simulink library "thc"  (R2021b)
settings: Solver=VariableStepAuto  StartTime=0.0  StopTime=10.0  RelTol=1e-3
undefined symbols (not defined in the file or in its folder): ATHC_APTCQA_X_C, ATHC_APTCQB_X_C, ATHC_dAy_X_C, ATHC_Qeq_X_kmh, ATHC_VbaseC_X_C, ATHC_VbaseC_Y_W, ATHC_VbaseD_X_C, ATHC_VbaseH_X_C, FALSE, KTHC_ACMaxMinT_sec, KTHC_aDeice_K, KTHC_AGSDefLv_K, KTHC_AGSLv1_K, KTHC_AGSLv2_K, KTHC_AGSLv3_K, KTHC_AGSLv4_K, KTHC_AGSLv5_K, KTHC_AirIntUpdateT_sec, KTHC_APTCOneZoneMax_W, KTHC_APTCPeriod_cnt, KTHC_APTCPWMEN_flg, KTHC_APTCQMaxC_W, KTHC_APTCQminC_W, KTHC_APTCQminD_W, KTHC_APTCQminRe1_W, KTHC_APTCQminRe_W, KTHC_APTCQoffT_cnt, KTHC_APTCQonT_cnt, KTHC_APTCRiLeMaxDff_W, KTHC_APTCRiLeMinDff_W, KTHC_BatInTempDef_C, KTHC_bDeice_K, KTHC_CompMaxDeice_rpm, KTHC_CompMinDeice_rpm, KTHC_CompSotxvOp_K, KTHC_CompSotxvOpLow_rpm, KTHC_CompSpdmax_rpm, KTHC_CompSpdmaxBC1_rpm, KTHC_CompSpdmaxBC_rpm, KTHC_CompSpdmid1_rpm, KTHC_CompSpdmid2_rpm, KTHC_CompSpdmid3_rpm, KTHC_CompSpdmid_rpm, KTHC_CompSpdmin_rpm, KTHC_DAPTCQ1_W, KTHC_DAPTCQ2_W, KTHC_DAPTCQ3_W, KTHC_DcChSetTemp_C, KTHC_DehumidityEN_flg, KTHC_DeiceCycTime_K, KTHC_DriveLevelWPTCBAH1_W, KTHC_DriveLevelWPTCBAH2_W, KTHC_DriveLevelWPTCBAH3_W, KTHC_DriveLevelWPTCBAH4_W, KTHC_DriveT1MinBAH_C, KTHC_DriveT2MaxBAH_C, KTHC_DriveT2MinBAH_C, KTHC_DriveT3MaxBAH_C, KTHC_DriveT3MinBAH_C, KTHC_DriveT4MaxBAH_C ... (+372)
libraries: simulink x140
(part 4 of 10)

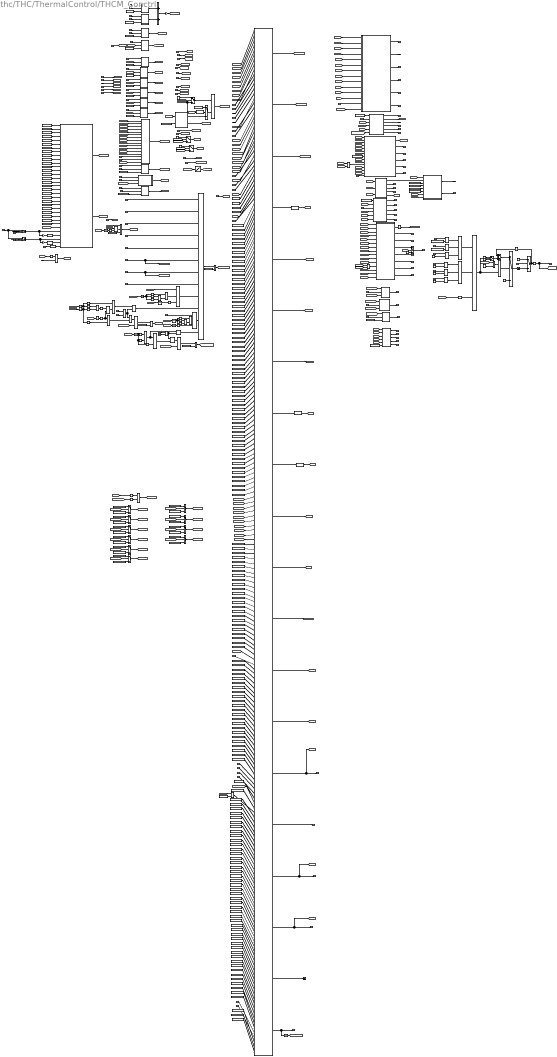
== system thc/THC/ThermalControl/THCM_Conctrl ==
  note: tick數 6000為10 min
  note: tick數 3000為5 min
  note: KTHC_DTcabin_C
  PwrSta : Inport
  AC : Inport  Port=2
  ACMax : Inport  Port=3
  ACAuto : Inport  Port=4
  sigSetTempZon1St : Inport  Port=5
  sigAirIntenZon1St : Inport  Port=6
  VehSpeed : Inport  Port=7
  HVBMTempMax : Inport  Port=8
  HVBMTempMin : Inport  Port=9
  OBCTemp : Inport  Port=10
  DCDCTemp : Inport  Port=11
  Rr_TMTemp : Inport  Port=12
  Rr_MCUTemp : Inport  Port=13
  Fr_TMTemp : Inport  Port=14
  Fr_MCUTemp : Inport  Port=15
  PT_ Low_P1 : Inport  Port=16
  PT_ Low_T1 : Inport  Port=17
  PT_Low_P2 : Inport  Port=18
  PT_ Low_T2 : Inport  Port=19
  PT_High_P : Inport  Port=20
  PT_High_Tact : Inport  Port=21
  Tamb : Inport  Port=22
  Bat_In_Temp : Inport  Port=23
  Bat_Out_Temp : Inport  Port=24
  Motor_In_Temp : Inport  Port=25
  Motor_Out_Temp : Inport  Port=26
  Tincar : Inport  Port=27
  SolarL : Inport  Port=28
  SolarR : Inport  Port=29
  Tevap : Inport  Port=30
  CompFB : Inport  Port=31
  CompProEN : Inport  Port=32
  VSCP_AGSCloseSta_flg : Inport  Port=33
  ShiftGearPosn : Inport  Port=34
  ChrgPlugSta : Inport  Port=35
  DfrstReq : Inport  Port=36
  WaterFillReq : Inport  Port=37
  sigSetTempZon2St : Inport  Port=38
  Fr_LLCTemp : Inport  Port=39
  Rr_LLCTemp : Inport  Port=40
  T_Face_L : Inport  Port=41
  T_Face_R : Inport  Port=42
  T_Foot_L : Inport  Port=43
  T_Foot_R : Inport  Port=44
  T_Face_Rr : Inport  Port=45
  T_Foot_Rr : Inport  Port=46
  PET : Inport  Port=47
  EACProtectEnable : Inport  Port=48
  Tamb_Err : Inport  Port=49
  SolarL_Err : Inport  Port=50
  SolarR_Err : Inport  Port=51
  Tevap_Err : Inport  Port=52
  T_Face_L_Err : Inport  Port=53
  T_Face_R_Err : Inport  Port=54
  T_Foot_L_Err : Inport  Port=55
  T_Foot_R_Err : Inport  Port=56
  T_Face_Rr_Err : Inport  Port=57
  T_Foot_Rr_Err : Inport  Port=58
  Tincar_Err : Inport  Port=59
  Bat_In_Temp_Err : Inport  Port=60
  Motor_In_Temp_Err : Inport  Port=61
  Motor_Out_Temp_Err : Inport  Port=62
  Fan_Err : Inport  Port=63
  AGS_Err : Inport  Port=64
  EWP3_Err : Inport  Port=65
  PT_High_P_Err : Inport  Port=66
  PT_High_Tact_Err : Inport  Port=67
  SOV1_Err : Inport  Port=68
  SOV2_Err : Inport  Port=69
  SOV3_Err : Inport  Port=70
  EXV1_Err : Inport  Port=71
  EXV2_Err : Inport  Port=72
  Comp_Err : Inport  Port=73
  Blower_Err : Inport  Port=74
  PT_Low_P1_Err : Inport  Port=75
  PT_Low_T1_Err : Inport  Port=76
  PT_Low_P2_Err : Inport  Port=77
  PT_Low_T2_Err : Inport  Port=78
  SOTXV_Err : Inport  Port=79
  ECOSW : Inport  Port=80
  RemoteACTemp : Inport  Port=81
  RemoteAutoReq : Inport  Port=82
  VINP_SmartEcoModeSW_flg : Inport  Port=83
  VINP_HVBIsoImpedenceN_Mohm : Inport  Port=84
  VINP_HVBIsoImpedenceP_Mohm : Inport  Port=85
  VINP_HVBHVILErr_flg : Inport  Port=86
  VINP_FrntPTCRearLeActHeatPwr_W : Inport  Port=87
  VINP_FrntPTCRearRiActHeatPwr_W : Inport  Port=88
  VINP_FrntPTCRiActHeatPwr_W : Inport  Port=89
  APTCFailDTC : Inport  Port=90
  RrAPTCEN : Inport  Port=91
  VINP_HVBattSOC_pct : Inport  Port=92
  VINP_IVIWPTCSWSta_flg : Inport  Port=93
  sigWindDirZon1St : Inport  Port=94
  1-D Lookup Table : Lookup_n-D  NumberOfTableDimensions=1  BreakpointsForDimension1=ATHC_dAy_X_C  Table=MTHC_dAy_Y_C  InternalRulePriority=Speed  RndMeth=Simplest  InputSameDT=on
  AGSandFan : Subsystem
  APTC : Subsystem
  Add1 : Sum
  Add2 : Sum
  BlowerCtrl : Subsystem
  Chart : Stateflow chart  TreatAsAtomicUnit=on
  Chart1 : Stateflow chart  TreatAsAtomicUnit=on
      settings: PortSchema="{\"entries\":[{\"content\":{\"sides\":[{\"content\":{\"connectorIds\":[\"In1\",\"In2\",\"In3\",\"In4\",\"In5\",\"In6\",\"In7\",\"In8\",\"In9\",\"In10\",\"In11\",\"In12\",\"In13\",\"In14\",\"In15\",\"In16\",\"In17\",\"In23\",\"In18\",\"In19\",\"In20\",\"In21\",\"In22\",\"In24\",\"In25\",\"In26\",\"In27\",\"In28\",\"In29\",\"In30\",\"In31\",\"In32\",\"In33\"]},\"type\":\"ConnectorPlacement.EquallySpacedRectSide\",\"uuid\":\"120e13ed-170d-4dd0-ac33-59229b58f73b\"},{\"content\":{\"connectorIds\":[\"Out1\",\"Out2\"],\"side\":\"RIGHT\"},\"type\":\"ConnectorPlacement.EquallySpacedRectSide\",\"uuid\":\"71523d45-f510-4724-888f-dcf7543ced53\"},{\"content\":{\"connectorIds\":[],\"side\":\"TOP\"},\"type\":\"ConnectorPlacement.EquallySpacedRectSide\",\"uuid\":\"9a401f36-06db-49d8-85fb-be71287fdb91\"}]},\"type\":\"ConnectorPlacement.EquallySpacedConnector\",\"uuid\":\"4c5defd4-093d-4cb1-85d3-718a50a7701f\"}],\"packageUris\":[\"http://schema.mathworks.com/mf0/Connector/R2020b\"],\"version\":\"1.0\"}"
  Chart2 : Stateflow chart  TreatAsAtomicUnit=on
  CompCtrl : Subsystem
  Compare To Constant : simulink/Logic and Bit Operations/Compare To Constant  relop=~=  const=1  OutDataTypeStr=boolean
  Compare To Constant1 : simulink/Logic and Bit Operations/Compare To Constant  relop=>  const=2  OutDataTypeStr=boolean
  Compare To Constant10 : simulink/Logic and Bit Operations/Compare To Constant  relop===  const=10  OutDataTypeStr=boolean
  Compare To Constant11 : simulink/Logic and Bit Operations/Compare To Constant  relop=~=  const=1  OutDataTypeStr=boolean
  Compare To Constant12 : simulink/Logic and Bit Operations/Compare To Constant  relop=>  const=2  OutDataTypeStr=boolean
  Compare To Constant13 : simulink/Logic and Bit Operations/Compare To Constant  relop=<  const=5  OutDataTypeStr=boolean
  Compare To Constant14 : simulink/Logic and Bit Operations/Compare To Constant  relop=<=  const=3.0  OutDataTypeStr=boolean
  Compare To Constant15 : simulink/Logic and Bit Operations/Compare To Constant  relop===  const=11  OutDataTypeStr=boolean
  Compare To Constant16 : simulink/Logic and Bit Operations/Compare To Constant  relop===  const=11  OutDataTypeStr=boolean
  Compare To Constant17 : simulink/Logic and Bit Operations/Compare To Constant  relop===  const=11  OutDataTypeStr=boolean
  Compare To Constant18 : simulink/Logic and Bit Operations/Compare To Constant  relop===  const=0  OutDataTypeStr=boolean
  Compare To Constant19 : simulink/Logic and Bit Operations/Compare To Constant  relop=>=  const=10  OutDataTypeStr=boolean
  Compare To Constant2 : simulink/Logic and Bit Operations/Compare To Constant  relop=<  const=10  OutDataTypeStr=boolean
  Compare To Constant20 : simulink/Logic and Bit Operations/Compare To Constant  relop=>  const=0  OutDataTypeStr=boolean
  Compare To Constant21 : simulink/Logic and Bit Operations/Compare To Constant  relop===  const=1  OutDataTypeStr=boolean
  Compare To Constant3 : simulink/Logic and Bit Operations/Compare To Constant  relop=>  const=7  OutDataTypeStr=boolean
  Compare To Constant4 : simulink/Logic and Bit Operations/Compare To Constant  relop=<  const=10  OutDataTypeStr=boolean
  Compare To Constant5 : simulink/Logic and Bit Operations/Compare To Constant  relop===  const=5  OutDataTypeStr=boolean
  Compare To Constant6 : simulink/Logic and Bit Operations/Compare To Constant  relop===  const=1  OutDataTypeStr=boolean
  Compare To Constant7 : simulink/Logic and Bit Operations/Compare To Constant  relop===  const=10  OutDataTypeStr=boolean
  Compare To Constant8 : simulink/Logic and Bit Operations/Compare To Constant  relop===  const=3  OutDataTypeStr=boolean
  Compare To Constant9 : simulink/Logic and Bit Operations/Compare To Constant  relop===  const=1  OutDataTypeStr=boolean
  Constant : Constant  Value=KTHC_T1MaxBC_C
  Constant1 : Constant  Value=KTHC_Plow2Setpoint_kPa
  Constant10 : Constant  Value=KTHC_T3MinBC_C
  Constant100 : Constant  Value=KTHC_Tdeheat2_C
  Constant101 : Constant  Value=KTHC_T1MinBAH_C
  Constant102 : Constant  Value=KTHC_CompMaxDeice_rpm
  Constant103 : Constant  Value=KTHC_CompMinDeice_rpm
  Constant104 : Constant  Value=KTHC_DeiceCycTime_K
  Constant105 : Constant  Value=KTHC_PDeiceMax_kPa
  Constant106 : Constant  Value=KTHC_TDeice1_C
  Constant107 : Constant  Value=KTHC_TDeice2_C
  Constant108 : Constant  Value=KTHC_TambHPmin_C
  Constant109 : Constant  Value=KTHC_Time0_K
  Constant11 : Constant  Value=KTHC_T3MaxBC_C
  Constant110 : Constant  Value=KTHC_TimeDeiceMax_K
  Constant111 : Constant  Value=KTHC_TwOhtOff_C
  Constant112 : Constant  Value=KTHC_TwOhtOn_C
  Constant113 : Constant  Value=KTHC_aDeice_K
  Constant114 : Constant  Value=KTHC_bDeice_K
  Constant115 : Constant  Value=KTHC_ta_K
  Constant116 : Constant  Value=KTHC_tb_K
  Constant117 : Constant  Value=KTHC_CompSotxvOpLow_rpm
  Constant118 : Constant  Value=KTHC_CompSotxvOp_K
  Constant119 : Constant  Value=KTHC_SotxvProHi_kPa
  Constant12 : Constant  Value=KTHC_T4MinBC_C
  Constant120 : Constant  Value=KTHC_SotxvProLo_kPa
  Constant121 : Constant  Value=KTHC_T1MaxLLC_C
  Constant122 : Constant  Value=KTHC_T2MinLLC_C
  Constant123 : Constant  Value=KTHC_T2MaxLLC_C
  Constant124 : Constant  Value=KTHC_T3MinLLC_C
  Constant125 : Constant  Value=KTHC_T3MaxLLC_C
  Constant126 : Constant  Value=KTHC_T4MinLLC_C
  Constant127 : Constant  Value=KTHC_T4MaxLLC_C
  Constant128 : Constant  Value=KTHC_T5MinLLC_C
  Constant129 : Constant  Value=KTHC_TDcChgBC_C
  Constant13 : Constant  Value=KTHC_EXV1SHSetpoint_K
  Constant130 : Constant  Value=KTHC_TambDef_C
  Constant131 : Constant  Value=KTHC_SolarDef_W
  Constant132 : Constant  Value=KTHC_SolarDef_W
  Constant133 : Constant  Value=KTHC_Tevap_C
  Constant{134..139} (6 alike) : Constant  Value=KTHC_TductDef_C
  Constant14 : Constant  Value=KTHC_T4MaxBC_C
  Constant140 : Constant  Value=KTHC_BatInTempDef_C
  Constant141 : Constant  Value=KTHC_MotorOutTempDef_C
  Constant142 : Constant  Value=KTHC_WPTCDef_W
  Constant143 : Constant  Value=KTHC_CompSpdmaxBC_rpm
  Constant{144..148} (5 alike) : Constant  Value=KTHC_ErrHandleEN_flg
  Constant149 : Constant  Value=17
  Constant15 : Constant  Value=KTHC_T5MinBC_C
  Constant150 : Constant  Value=32
  Constant151 : Constant  Value=32
  Constant152 : Constant  Value=KTHC_SolarDebounceT_sec
  Constant153 : Constant  Value=KTHC_DTcabin_C
  Constant154 : Constant  Value=KTHC_DTreturn1_C
  Constant155 : Constant  Value=KTHC_DTreturn_C
  Constant156 : Constant  Value=KTHC_ECOTambLV1_C
  Constant157 : Constant  Value=KTHC_ECOTambLV2_C
  Constant158 : Constant  Value=KTHC_ECOTambLV3_C
  Constant159 : Constant  Value=KTHC_ECOTambLV4_C
  Constant16 : Constant  Value=KTHC_T1MaxCCU_C
  Constant160 : Constant  Value=KTHC_ECOTambLVT_sec
  Constant161 : Constant  Value=KTHC_ECOalpha1_K
  Constant162 : Constant  Value=KTHC_ECOalpha2_K
  Constant163 : Constant  Value=KTHC_ECOalpha3_K
  Constant164 : Constant  Value=KTHC_ECOalpha4_K
  Constant165 : Constant  Value=KTHC_ECOalpha5_K
  Constant166 : Constant  Value=KTHC_ECObeta1_K
  Constant167 : Constant  Value=KTHC_ECObeta2_K
  Constant168 : Constant  Value=KTHC_ECObeta3_K
  Constant169 : Constant  Value=KTHC_ECObeta4_K
  Constant17 : Constant  Value=KTHC_T3MinCCU_C
  Constant170 : Constant  Value=KTHC_ECObeta5_K
  Constant171 : Constant  Value=KTHC_ECObeta6_K
  Constant172 : Constant  Value=KTHC_ECObeta7_K
  Constant173 : Constant  Value=KTHC_ECObeta8_K
  Constant174 : Constant  Value=KTHC_ECObeta9_K
  Constant175 : Constant  Value=KTHC_ECOalpha6_K
  Constant176 : Constant  Value=KTHC_ECOalpha7_K
  Constant177 : Constant  Value=KTHC_ECOalpha8_K
  Constant178 : Constant  Value=KTHC_ECOalpha9_K
  Constant179 : Constant  Value=KTHC_ECOTambLV5_C
  Constant18 : Constant  Value=KTHC_T3MaxCCU_C
  Constant180 : Constant  Value=KTHC_ECOTambLV6_C
  Constant181 : Constant  Value=KTHC_ECOTambLV7_C
  Constant182 : Constant  Value=KTHC_ECOTambLV8_C
  Constant183 : Constant  Value=KTHC_DTcabin1_C
  Constant184 : Constant  Value=KTHC_DTcabin2_C
  Constant185 : Constant  Value=KTHC_DTreturn3_C
  Constant186 : Constant  Value=KTHC_DTimeCD_K
  Constant187 : Constant  Value=KTHC_DTambSat1_C
  Constant188 : Constant  Value=KTHC_DTambSat2_C
  Constant189 : Constant  Value=KTHC_APTCQMaxC_W
  Constant19 : Constant  Value=KTHC_T4MinCCU_C
  Constant190 : Constant  Value=KTHC_DTreturn2_C
  Constant191 : Constant  Value=KTHC_DTcabin3_C
  Constant192 : Constant  Value=KTHC_DTcabin4_C
  Constant193 : Constant  Value=KTHC_DTcabin5_C
  Constant194 : Constant  Value=KTHC_DTcabin6_C
  Constant195 : Constant  Value=KTHC_DTimeCD1_K
  Constant196 : Constant  Value=KTHC_DTimeCD2_K
  Constant197 : Constant  Value=KTHC_TambACmode1_C
  Constant198 : Constant  Value=KTHC_TambACmode2_C
  Constant199 : Constant  Value=KTHC_TambACmode3_C
  Constant2 : Constant  Value=KTHC_Timehu1_K
  Constant20 : Constant  Value=KTHC_T4MaxCCU_C
  Constant200 : Constant  Value=KTHC_TambACmode4_C
  Constant201 : Constant  Value=KTHC_DTcabin7_C
  Constant202 : Constant  Value=KTHC_DTcabin9_C
  Constant203 : Constant  Value=KTHC_DTcabin10_C
  Constant204 : Constant  Value=KTHC_DTreturn6_C
  Constant205 : Constant  Value=KTHC_DTambSat5_C
  Constant206 : Constant  Value=KTHC_APTCQminRe1_W
  Constant207 : Constant  Value=KTHC_DTCabin11_C
  Constant208 : Constant  Value=KTHC_TambSetLow_C
  Constant209 : Constant  Value=KTHC_Tcoolmin_C
  Constant21 : Constant  Value=KTHC_T5MinCCU_C
  Constant210 : Constant  Value=KTHC_TimeRe1_sec
  Constant211 : Constant  Value=KTHC_TimeRe2_sec
  Constant212 : Constant  Value=KTHC_Trecymin_C
  Constant213 : Constant  Value=KTHC_WoWPTC_flg
  Constant214 : Constant  Value=KTHC_DTreturn7_C
  Constant215 : Constant  Value=KTHC_DTambsat3_C
  Constant216 : Constant  Value=KTHC_TambACmode5_C
  Constant217 : Constant  Value=KTHC_TambACmode6_C
  Constant218 : Constant  Value=KTHC_CompSpdmid1_rpm
  Constant219 : Constant  Value=KTHC_CompSpdmid2_rpm
  Constant22 : Constant  Value=KTHC_T2MinCCU_C
  Constant220 : Constant  Value=KTHC_CompSpdmid3_rpm
  Constant221 : Constant  Value=KTHC_DTcabin12_C
  Constant222 : Constant  Value=KTHC_CompSpdmaxBC1_rpm
  Constant223 : Constant  Value=KTHC_HVBIsoImpedenceLV_Mohm
  Constant224 : Constant  Value=KTHC_HVBIsoImpedenceLV_Mohm
  Constant{225..228,244} (5 alike) : Constant  Value=0
  Constant229 : Constant  Value=KTHC_DriveT1MinBAH_C
  Constant23 : Constant  Value=KTHC_T2MaxCCU_C
  Constant230 : Constant  Value=KTHC_T2MinBAH_C
  Constant231 : Constant  Value=KTHC_DriveT2MinBAH_C
  Constant232 : Constant  Value=KTHC_DriveT3MaxBAH_C
  Constant233 : Constant  Value=KTHC_DTambsat4_C
  Constant234 : Constant  Value=KTHC_TambACmode7_C
  Constant235 : Constant  OutDataTypeStr=uint8
  Constant236 : Constant  Value=0  OutDataTypeStr=uint8
  Constant237 : Constant  Value=0  OutDataTypeStr=uint8
  Constant238 : Constant  Value=0  OutDataTypeStr=uint8
  Constant239 : Constant  Value=10  OutDataTypeStr=uint8
  Constant24 : Constant  Value=KTHC_T1MaxMCU_C
  Constant240 : Constant  Value=KTHC_DriveT2MaxBAH_C
  Constant241 : Constant  Value=KTHC_DriveT4MaxBAH_C
  Constant242 : Constant  Value=KTHC_LevelWPTCBAH3_W
  Constant243 : Constant  Value=KTHC_DriveLevelWPTCBAH1_W
  Constant245 : Constant  Value=KTHC_LevelWPTCBAH4_W
  Constant246 : Constant  Value=KTHC_DriveLevelWPTCBAH4_W
  Constant247 : Constant  Value=KTHC_EWPBalanceSW_flg
  Constant248 : Constant  Value=KTHC_DTwBMoin3_C
  Constant249 : Constant  Value=KTHC_HeatingFactor_C
  Constant25 : Constant  Value=KTHC_T3MinMCU_C
  Constant250 : Constant  Value=KTHC_ForceLeaveCool_C
  Constant251 : Constant  Value=KTHC_ForceLeaveHeat_C
  Constant26 : Constant  Value=KTHC_T3MaxMCU_C
  Constant27 : Constant  Value=KTHC_T4MinMCU_C
  Constant28 : Constant  Value=KTHC_T4MaxMCU_C
  Constant29 : Constant  Value=KTHC_T5MinMCU_C
  Constant3 : Constant  Value=KTHC_Timehu2_K
  Constant30 : Constant  Value=KTHC_T2MinMCU_C
  Constant31 : Constant  Value=KTHC_T2MaxMCU_C
  Constant32 : Constant  Value=KTHC_T1MaxMT_C
  Constant33 : Constant  Value=KTHC_T3MinMT_C
  Constant34 : Constant  Value=KTHC_T3MaxMT_C
  Constant35 : Constant  Value=KTHC_T4MinMT_C
  Constant36 : Constant  Value=KTHC_T4MaxMT_C
  Constant37 : Constant  Value=KTHC_T5MinMT_C
  Constant38 : Constant  Value=KTHC_T2MinMT_C
  Constant39 : Constant  Value=KTHC_T2MaxMT_C
  Constant4 : Constant  Value=KTHC_EXV2SHSetpoint_K
  Constant40 : Constant  Value=KTHC_P3MinHi_kPa
  Constant41 : Constant  Value=KTHC_P3MaxHi_kPa
  Constant42 : Constant  Value=KTHC_P4MinHi_kPa
  Constant43 : Constant  Value=KTHC_P4MaxHi_kPa
  Constant44 : Constant  Value=KTHC_P5MinHi_kPa
  Constant45 : Constant  Value=KTHC_P2MaxHi_kPa
  Constant46 : Constant  Value=KTHC_P3MaxLo_kPa
  Constant47 : Constant  Value=KTHC_P3MinLo_kPa
  Constant48 : Constant  Value=KTHC_P4MaxLo_kPa
  Constant49 : Constant  Value=KTHC_P4MinLo_kPa
  Constant5 : Constant  Value=KTHC_Tice_C
  Constant50 : Constant  Value=KTHC_P5MaxLo_kPa
  Constant51 : Constant  Value=KTHC_P2MinLo_kPa
  Constant52 : Constant  Value=KTHC_TWVRcolPos_pct
  Constant53 : Constant  Value=KTHC_TwRcolOn_C
  Constant54 : Constant  Value=KTHC_TwRcolOff_C
  Constant55 : Constant  Value=KTHC_DTambSat_C
  Constant56 : Constant  Value=KTHC_VehSdFanOn_kph
  Constant57 : Constant  Value=KTHC_VehSdFanOff_kph
  Constant58 : Constant  Value=KTHC_VehSdAGS100_kph
  Constant59 : Constant  Value=KTHC_VehSdAGSCtrl_kph
  Constant6 : Constant  Value=KTHC_Tdeice_C
  Constant60 : Constant  Value=KTHC_T2MinBH_C
  Constant61 : Constant  Value=KTHC_T3MaxBH_C
  Constant62 : Constant  Value=KTHC_T3MinBH_C
  Constant63 : Constant  Value=KTHC_T4MaxBH_C
  Constant64 : Constant  Value=KTHC_T4MinBH_C
  Constant65 : Constant  Value=KTHC_T5MaxBH_C
  Constant66 : Constant  Value=KTHC_DriveT3MinBAH_C
  Constant67 : Constant  Value=KTHC_T3MaxBAH_C
  Constant68 : Constant  Value=KTHC_T3MinBAH_C
  Constant69 : Constant  Value=KTHC_T4MaxBAH_C
  Constant7 : Constant  Value=KTHC_APTCQminD_W
  Constant70 : Constant  Value=KTHC_T2MaxBAH_C
  Constant71 : Constant  Value=KTHC_LevelWPTCBAH1_W
  Constant72 : Constant  Value=KTHC_DriveLevelWPTCBAH2_W
  Constant73 : Constant  Value=KTHC_LevelWPTCBAH2_W
  Constant74 : Constant  Value=KTHC_TWinmax_C
  Constant75 : Constant  Value=KTHC_TWinmin_C
  Constant76 : Constant  Value=KTHC_DriveLevelWPTCBAH3_W
  Constant77 : Constant  Value=KTHC_T1MinBH_C
  Constant78 : Constant  Value=KTHC_T2MaxBH_C
  Constant79 : Constant  Value=KTHC_DTwBMoin1_C
  Constant8 : Constant  Value=KTHC_T2MinBC_C
  Constant80 : Constant  Value=KTHC_DTwBMoin2_C
  Constant81 : Constant  Value=KTHC_DTwBBin_C
  Constant82 : Constant  Value=KTHC_CompSpdmax_rpm
  Constant83 : Constant  Value=KTHC_TBPmax_C
  Constant84 : Constant  Value=KTHC_TBPmin_C
  Constant85 : Constant  Value=KTHC_T3winSetpointBC_C
  Constant86 : Constant  Value=KTHC_Timewcd_K
  Constant87 : Constant  Value=KTHC_CompSpdmin_rpm
  Constant88 : Constant  Value=KTHC_Plow2Setpoint_kPa
  Constant89 : Constant  Value=KTHC_DTh1_C
  Constant9 : Constant  Value=KTHC_T2MaxBC_C
  Constant90 : Constant  Value=KTHC_Tambset_C
  Constant91 : Constant  Value=KTHC_Twmset_C
  Constant92 : Constant  Value=KTHC_APTCQminRe_W
  Constant93 : Constant  Value=KTHC_CompSpdmid_rpm
  Constant94 : Constant  Value=KTHC_PhiDehum_kPa
  Constant95 : Constant  Value=KTHC_ThiDehum_C
  Constant96 : Constant  Value=KTHC_DehumidityEN_flg
  Constant97 : Constant  Value=KTHC_TimeD_K
  Constant98 : Constant  Value=KTHC_Tdefog_C
  Constant99 : Constant  Value=KTHC_Tdeheat1_C
  Data Type Conversion : DataTypeConversion  OutDataTypeStr=uint16
  Data Type Conversion1 : DataTypeConversion  OutDataTypeStr=uint16
  Data Type Conversion2 : DataTypeConversion  OutDataTypeStr=boolean
  EWP1 : Subsystem
  EWP2 : Subsystem
  EWP3 : Subsystem
  EXV1Ctrl : Subsystem
  EXV2Ctrl : Subsystem
  Gain : Gain  Gain=10
  Gain1 : Gain  Gain=10
  Gain2 : Gain  Gain=1/2
  Logical Operator{,12..13,31} (4 alike) : Logic  Inputs=3  AllPortsSameDT=off  OutDataTypeStr=boolean
  Logical Operator{1,3..5,10,14,17..18,25,27..28,32..33} (13 alike) : Logic  Operator=OR  AllPortsSameDT=off  OutDataTypeStr=boolean
  Logical Operator{2,6..7,9,11,15..16,19..24,26,35} (15 alike) : Logic  AllPortsSameDT=off  OutDataTypeStr=boolean
  Logical Operator29 : Logic  Operator=OR  Inputs=3  AllPortsSameDT=off  OutDataTypeStr=boolean
  Logical Operator30 : Logic  Operator=OR  Inputs=3  AllPortsSameDT=off  OutDataTypeStr=boolean
  Logical Operator8 : Logic  Operator=OR  Inputs=12  AllPortsSameDT=off  OutDataTypeStr=boolean
  NOT : Logic  Operator=NOT  IconShape=distinctive  AllPortsSameDT=off  OutDataTypeStr=boolean
  Product : Product
  RadiatorFan : Subsystem
  Relational Operator : RelationalOperator  Operator=<=  OutDataTypeStr=boolean  RndMeth=Simplest
  Relational Operator1 : RelationalOperator  Operator=<=  OutDataTypeStr=boolean  RndMeth=Simplest
  Relational Operator2 : RelationalOperator  Operator=~=  OutDataTypeStr=boolean  RndMeth=Simplest
  Relational Operator{3..5,7} (4 alike) : RelationalOperator  Operator=>  OutDataTypeStr=boolean  RndMeth=Simplest
  Saturation1 : Saturate  UpperLimit=10  LowerLimit=0
  Scope : Scope
  SensorErrorHandle1 : Subsystem
  SensorErrorHandle10 : Subsystem
  SensorErrorHandle11 : Subsystem
  SensorErrorHandle12 : Subsystem
  SensorErrorHandle2 : Subsystem
  SensorErrorHandle3 : Subsystem
  SensorErrorHandle4 : Subsystem
  SensorErrorHandle5 : Subsystem
  SensorErrorHandle6 : Subsystem
  SensorErrorHandle7 : Subsystem
  SensorErrorHandle8 : Subsystem
  SensorErrorHandle9 : Subsystem
  Subsystem : Subsystem
  Subsystem1 : Subsystem
  Subsystem2 : Subsystem
  Subsystem3 : Subsystem
  Subsystem4 : Subsystem
  Switch{,1..19} (20 alike) : Switch  Criteria=u2 > Threshold
  Thermal : Stateflow chart  TreatAsAtomicUnit=on
      settings: PortSchema="{\"entries\":[{\"content\":{\"sides\":[{\"content\":{\"connectorIds\":[\"In22\",\"In1\",\"In2\",\"In3\",\"In4\",\"In5\",\"In6\",\"In7\",\"In8\",\"In9\",\"In10\",\"In11\",\"In12\",\"In13\",\"In14\",\"In15\",\"In18\",\"In16\",\"In17\",\"In19\",\"In20\",\"In21\",\"In23\",\"In24\",\"In25\",\"In26\",\"In27\",\"In28\",\"In29\",\"In30\",\"In31\",\"In32\",\"In33\",\"In34\",\"In35\",\"In36\",\"In37\",\"In38\",\"In39\",\"In40\",\"In41\",\"In42\",\"In43\",\"In44\",\"In45\",\"In46\",\"In47\",\"In48\",\"In49\",\"In50\",\"In51\",\"In52\",\"In53\",\"In54\",\"In55\",\"In56\",\"In57\",\"In58\",\"In59\",\"In60\",\"In61\",\"In62\",\"In63\",\"In64\",\"In65\",\"In66\",\"In67\",\"In68\",\"In69\",\"In70\",\"In71\",\"In72\",\"In73\",\"In74\",\"In75\",\"In76\",\"In77\",\"In78\",\"In79\",\"In80\",\"In81\",\"In82\",\"In83\",\"In84\",\"In85\",\"In86\",\"In87\",\"In88\",\"In89\",\"In90\",\"In91\",\"In92\",\"In93\",\"In94\",\"In95\",\"In96\",\"In97\",\"In137\",\"In98\",\"In99\",\"In100\",\"In101\",\"In102\",\"In103\",\"In104\",\"In105\",\"In106\",\"In107\",\"In108\",\"In109\",\"In110\",\"In111\",\"In112\",\"In113\",\"In114\",\"In115\",\"In116\",\"In117\",\"In118\",\"In119\",\"In120\",\"In121\",\"In122\",\"In123\",\"In124\",\"In125\",\"In126\",\"In127\",\"In128\",\"In129\",\"In130\",\"In131\",\"In132\",\"In133\",\"In134\",\"In135\",\"In136\",\"In138\",\"In139\",\"In140\",\"In141\",\"In142\",\"In143\",\"In144\",\"In145\",\"In146\",\"In147\",\"In148\",\"In149\",\"In150\",\"In151\",\"In152\",\"In153\",\"In154\",\"In155\",\"In156\",\"In157\",\"In158\",\"In159\",\"In160\",\"In161\",\"In162\",\"In163\",\"In164\",\"In165\",\"In166\",\"In167\",\"In168\",\"In169\",\"In170\",\"In171\",\"In172\",\"In173\",\"In174\",\"In175\",\"In176\",\"In177\",\"In178\",\"In179\",\"In180\",\"In181\",\"In182\",\"In183\",\"In184\",\"In185\",\"In186\",\"In187\",\"In188\",\"In189\",\"In190\",\"In191\",\"In192\",\"In193\",\"In194\",\"In195\",\"In196\",\"In197\",\"In198\",\"In199\",\"In200\",\"In201\",\"In202\",\"In203\",\"In204\",\"In205\",\"In206\",\"In207\",\"In208\",\"In209\",\"In210\",\"In211\",\"In212\",\"In213\",\"In214\"]},\"type\":\"ConnectorPlacement.EquallySpacedRectSide\",\"uuid\":\"f0032f37-379c-4410-84d7-1f2e4d737994\"},{\"content\":{\"connectorIds\":[\"Out1\",\"Out2\",\"Out3\",\"Out4\",\"Out5\",\"Out6\",\"Out7\",\"Out8\",\"Out9\",\"Out10\",\"Out11\",\"Out12\",\"Out13\",\"Out14\",\"Out16\",\"Out18\",\"Out17\",\"Out15\",\"Out19\",\"Out20\"],\"side\":\"RIGHT\"},\"type\":\"ConnectorPlacement.EquallySpacedRectSide\",\"uuid\":\"1de0eec4-8da4-4f67-b701-80b707ee0866\"},{\"content\":{\"connectorIds\":[],\"side\":\"TOP\"},\"type\":\"ConnectorPlacement.EquallySpacedRectSide\",\"uuid\":\"b83953a5-08e8-430f-9593-9d2c74d0a81a\"}]},\"type\":\"ConnectorPlacement.EquallySpacedConnector\",\"uuid\":\"ef17bb72-69cc-4173-9cd7-5d5a49851498\"}],\"packageUris\":[\"http://schema.mathworks.com/mf0/Connector/R2020b\"],\"version\":\"1.0\"}"
  Unit Delay{,1..11} (12 alike) : UnitDelay  SampleTime=-1  HasFrameUpgradeWarning=on
  WPTC : Subsystem
  FD_Comp_Cmd : Outport
  FD_SOV1_Cmd : Outport  Port=2
  FD_SOV2_Cmd : Outport  Port=3
  FD_SOV3_Cmd : Outport  Port=4
  FD_EXV1_Cmd : Outport  Port=5
  FD_EXV2_Cmd : Outport  Port=6
  FD_SOTXV_Cmd : Outport  Port=7
  FD_FWV_Cmd : Outport  Port=8
  FD_TWV_Cmd : Outport  Port=9
  FD_FrWPTCHeatPwr_Cmd : Outport  Port=10
  CoolgFanActDuty : Outport  Port=11
  FD_AGS_Cmd : Outport  Port=12
  FD_EWP1_Cmd : Outport  Port=13
  FD_EWP2_Cmd : Outport  Port=14
  FD_EWP3_Cmd : Outport  Port=15
  FD_FrLeAPTCHeatPwr_Cmd : Outport  Port=16
  FD_FrRiAPTCHeatPwr_Cmd : Outport  Port=17
  FD_RrAPTCHeatPwr_Cmd : Outport  Port=18
  FD_Blower_Cmd : Outport  Port=19
  BatteryMode : Outport  Port=20
  EDriveMode : Outport  Port=21
  CabinMode : Outport  Port=22
  ACSubMode : Outport  Port=23
  VTHC_CompP_K : Outport  Port=24
  VTHC_CompI_K : Outport  Port=25
  VTHC_CompU_K : Outport  Port=26
  VTHC_CompDeltaU_K : Outport  Port=27
  VTHC_Compe_K : Outport  Port=28
  VTHC_Blowere_K : Outport  Port=29
  VTHC_BlowerP_K : Outport  Port=30
  VTHC_BlowerU_K : Outport  Port=31
  VTHC_Vbase_pct : Outport  Port=32
  VTHC_BlowerI_K : Outport  Port=33
  VTHC_EXV2P_K : Outport  Port=34
  VTHC_EXV2I_K : Outport  Port=35
  VTHC_EXV2U_K : Outport  Port=36
  VTHC_EXV2e_K : Outport  Port=37
  VTHC_APTCP_K : Outport  Port=38
  VTHC_APTCI_K : Outport  Port=39
  VTHC_APTCU_K : Outport  Port=40
  VTHC_APTCe_K : Outport  Port=41
  VTHC_EXV1P_K : Outport  Port=42
  VTHC_EXV1I_K : Outport  Port=43
  VTHC_EXV1U_K : Outport  Port=44
  VTHC_EXV1e_K : Outport  Port=45
  VTHC_FDCTHCMAPTCForceOFFSta_flg : Outport  Port=46
  VTHC_FDCTHCMPreWPTCHeatSta_enum : Outport  Port=47
  wires:
  Constant234/1 -> Thermal/209(KTHC_TambACmode7_C)
  Constant233/1 -> Thermal/208(KTHC_DTambsat4_C)
  [APTCForceOFF] -> Logical Operator33/2
  [ErrAPTCForceOFF] -> Logical Operator33/1
  Logical Operator33/1 -> APTC/12(ErrAPTCForceOFF)
  Logical Operator30/1 -> Logical Operator31/2
  Logical Operator29/1 -> Logical Operator31/1
  Relational Operator5/1 -> Logical Operator30/3
  Relational Operator4/1 -> Logical Operator30/2
  Relational Operator3/1 -> Logical Operator30/1
  Constant228/1 -> Relational Operator5/2
  VINP_FrntPTCRiActHeatPwr_W/1 -> Relational Operator5/1
  VINP_FrntPTCRearRiActHeatPwr_W/1 -> Relational Operator4/1
  Constant227/1 -> Relational Operator4/2
  Constant226/1 -> Relational Operator3/2
  VINP_FrntPTCRearLeActHeatPwr_W/1 -> Relational Operator3/1
  Relational Operator/1 -> Logical Operator29/1
  Relational Operator1/1 -> Logical Operator29/2
  Relational Operator2/1 -> Logical Operator29/3
  Constant225/1 -> Relational Operator2/2
  VINP_HVBHVILErr_flg/1 -> Relational Operator2/1
  Constant224/1 -> Relational Operator1/2
  VINP_HVBIsoImpedenceP_Mohm/1 -> Relational Operator1/1
  Constant223/1 -> Relational Operator/2
  VINP_HVBIsoImpedenceN_Mohm/1 -> Relational Operator/1
  Constant222/1 -> Thermal/207(KTHC_CompSpdmaxBC1_rpm)
  VINP_SmartEcoModeSW_flg/1 -> CompCtrl/15(VINP_SmartEcoModeSW_flg)
  Constant221/1 -> Thermal/206(KTHC_DTcabin12_C)
  Constant220/1 -> Thermal/205(KTHC_CompSpdmid3_rpm)
  Constant219/1 -> Thermal/204(KTHC_CompSpdmid2_rpm)
  Constant218/1 -> Thermal/203(KTHC_CompSpdmid1_rpm)
  [ACSubMode] -> Subsystem1/16(ACSubMode)
  Compare To Constant17/1 -> Logical Operator28/2
  Unit Delay9/1 -> Compare To Constant17/1
  [CabinMode] -> Unit Delay9/1
  Logical Operator28/1 -> Logical Operator13/2
  [AC] -> Logical Operator28/1
  Logical Operator27/1 -> Logical Operator12/2
  Compare To Constant16/1 -> Logical Operator27/1
  Logical Operator26/1 -> Logical Operator27/2
  Logical Operator25/1 -> Logical Operator/2
  Compare To Constant15/1 -> Logical Operator25/1
  Logical Operator24/1 -> Logical Operator25/2
  Constant217/1 -> Thermal/202(KTHC_TambACmode6_C)
  Constant216/1 -> Thermal/201(KTHC_TambACmode5_C)
  Constant215/1 -> Thermal/200(KTHC_DTambsat3_C)
  Constant214/1 -> Thermal/199(KTHC_DTreturn7_C)
  [PT_Low_P1] -> CompCtrl/14(PT_Low_P1)
  Constant213/1 -> Thermal/198(KTHC_WoWPTC_flg)
  [AC] -> APTC/15(AC)
  Data Type Conversion2/1 -> Chart1/33(ECOSW)
  Constant212/1 -> Thermal/197(KTHC_Trecymin_C)
  Constant211/1 -> Thermal/196(KTHC_TimeRe2_sec)
  Constant210/1 -> Thermal/195(KTHC_TimeRe1_sec)
  Constant209/1 -> Thermal/194(KTHC_Tcoolmin_C)
  Constant208/1 -> Thermal/193(KTHC_TambSetLow_C)
  Constant207/1 -> Thermal/192(KTHC_DTCabin11_C)
  Constant206/1 -> Thermal/191(KTHC_APTCQminRe1_W)
  [Tamb] -> APTC/14(Tamb)
  Constant205/1 -> Thermal/190(KTHC_DTambSat5_C)
  Constant204/1 -> Thermal/189(KTHC_DTreturn6_C)
  Constant203/1 -> Thermal/188(KTHC_DTcabin10_C)
  Constant202/1 -> Thermal/187(KTHC_DTcabin9_C)
  Thermal/1(AGS) -> [AGS]
  sigSetTempZon2St/1 -> Switch4/3
  sigSetTempZon1St/1 -> Switch3/3
  RemoteACTemp/1 -> Switch4/1, Switch3/1
  [Remote_AutoReq] -> Switch3/2
  [Remote_AutoReq] -> Switch4/2
  Compare To Constant14/1 -> Logical Operator23/1
  [PwrSta] -> Compare To Constant14/1
  Logical Operator23/1 -> [Remote_AutoReq]
  RemoteAutoReq/1 -> Logical Operator23/2
  Data Type Conversion1/1 -> Chart1/32(SetTempZon2St_CMD)
  Switch4/1 -> Chart1/31(sigSetTempZon2St), Gain1/1
  Gain1/1 -> Data Type Conversion1/1
  Data Type Conversion/1 -> Chart1/30(SetTempZon1St_CMD)
  Gain/1 -> Data Type Conversion/1
  Constant201/1 -> Thermal/186(KTHC_DTcabin7_C)
  Constant200/1 -> Thermal/185(KTHC_TambACmode4_C)
  Constant199/1 -> Thermal/184(KTHC_TambACmode3_C)
  Constant198/1 -> Thermal/183(KTHC_TambACmode2_C)
  Constant197/1 -> Thermal/182(KTHC_TambACmode1_C)
  Constant196/1 -> Thermal/181(KTHC_DTimeCD2_K)
  Constant195/1 -> Thermal/180(KTHC_DTimeCD1_K)
  Constant194/1 -> Thermal/179(KTHC_DTcabin6_C)
  Constant193/1 -> Thermal/178(KTHC_DTcabin5_C)
  Constant192/1 -> Thermal/177(KTHC_DTcabin4_C)
  Constant191/1 -> Thermal/176(KTHC_DTcabin3_C)
  Constant190/1 -> Thermal/175(KTHC_DTreturn2_C)
  Constant189/1 -> Thermal/174(KTHC_APTCQMaxC_W)
  [sigSetTempZon1StC] -> APTC/13(sigSetTempZon1StC)
  Constant188/1 -> Thermal/173(KTHC_DTambSat2_C)
  Constant187/1 -> Thermal/172(KTHC_DTambSat1_C)
  Constant185/1 -> Thermal/170(KTHC_DTreturn3_C)
  Constant186/1 -> Thermal/171(KTHC_DTimeCD_K)
  Constant184/1 -> Thermal/169(KTHC_DTcabin2_C)
  Constant183/1 -> Thermal/168(KTHC_DTcabin1_C)
  Constant182/1 -> Chart1/8(KTHC_ECOTambLV8_C)
  Constant181/1 -> Chart1/7(KTHC_ECOTambLV7_C)
  Constant180/1 -> Chart1/6(KTHC_ECOTambLV6_C)
  Constant179/1 -> Chart1/5(KTHC_ECOTambLV5_C)
  Constant178/1 -> Chart1/23(KTHC_ECOalpha9_K)
  Constant177/1 -> Chart1/17(KTHC_ECOalpha8_K)
  Constant176/1 -> Chart1/16(KTHC_ECOalpha7_K)
  Constant175/1 -> Chart1/15(KTHC_ECOalpha6_K)
  Constant174/1 -> Chart1/27(KTHC_ECObeta9_K)
  Constant173/1 -> Chart1/26(KTHC_ECObeta8_K)
  Constant172/1 -> Chart1/25(KTHC_ECObeta7_K)
  Constant171/1 -> Chart1/24(KTHC_ECObeta6_K)
  [sigSetTempZon2Stadj] -> Switch2/3
  [sigSetTempZon1Stadj] -> Switch1/3
  Chart1/2(sigSetTempZon2Stadj) -> [sigSetTempZon2Stadj]
  Chart1/1(sigSetTempZon1Stadj) -> [sigSetTempZon1Stadj]
  Constant170/1 -> Chart1/22(KTHC_ECObeta5_K)
  Constant169/1 -> Chart1/21(KTHC_ECObeta4_K)
  Constant168/1 -> Chart1/20(KTHC_ECObeta3_K)
  Constant167/1 -> Chart1/19(KTHC_ECObeta2_K)
  Constant166/1 -> Chart1/18(KTHC_ECObeta1_K)
  Constant165/1 -> Chart1/14(KTHC_ECOalpha5_K)
  Constant164/1 -> Chart1/13(KTHC_ECOalpha4_K)
  Constant163/1 -> Chart1/12(KTHC_ECOalpha3_K)
  Constant162/1 -> Chart1/11(KTHC_ECOalpha2_K)
  Constant161/1 -> Chart1/10(KTHC_ECOalpha1_K)
  Constant160/1 -> Chart1/9(KTHC_ECOTambLVT_sec)
  Constant159/1 -> Chart1/4(KTHC_ECOTambLV4_C)
  Constant158/1 -> Chart1/3(KTHC_ECOTambLV3_C)
  Constant157/1 -> Chart1/2(KTHC_ECOTambLV2_C)
  Constant156/1 -> Chart1/1(KTHC_ECOTambLV1_C)
  ECOSW/1 -> Data Type Conversion2/1
  [Tamb] -> Chart1/28(Tamb)
  Switch3/1 -> Chart1/29(sigSetTempZon1St), Gain/1
  Constant155/1 -> Thermal/167(KTHC_DTreturn_C)
  Constant154/1 -> Thermal/166(KTHC_DTreturn1_C)
  Constant153/1 -> Thermal/165(KTHC_DTcabin_C)
  Chart2/2(Blowersolar) -> [Blowersolar]
  Constant152/1 -> Chart2/2(KTHC_SolarDebounceT_sec)
  [sigSetTempZon2St] -> APTC/5(sigSetTempZon2St)
  [ACMax] -> Switch2/2
  Switch2/1 -> [sigSetTempZon2St]
  Constant151/1 -> Switch2/1
  Constant150/1 -> Switch1/1
  Switch1/1 -> [sigSetTempZon1St]
  [ACMax] -> Switch1/2
  Constant149/1 -> Switch/1
  [ACMax] -> Switch/2
  Switch/1 -> Product/1
  [sigSetTempZon1St] -> Subsystem4/1(sigSetTempZon1St), Switch/3
  [ACMax] -> Thermal/1(ACMax)
  ACMax/1 -> [ACMax]
  [Tamb_Err] -> Logical Operator22/1
  Logical Operator22/1 -> Thermal/164(Tamb_Err)
  Constant148/1 -> Logical Operator22/2
  Logical Operator21/1 -> [ErrEXV2FroceOFF]
  Logical Operator18/1 -> Logical Operator21/1
  Constant147/1 -> Logical Operator21/2
  Logical Operator17/1 -> Logical Operator20/1
  Logical Operator20/1 -> [ErrEXV1FroceOFF]
  Constant146/1 -> Logical Operator20/2
  Constant145/1 -> Logical Operator13/3
  Logical Operator8/1 -> Logical Operator19/1
  Logical Operator19/1 -> [ErrCompForceOFF]
  Constant144/1 -> Logical Operator19/2
  [Tamb] -> CompCtrl/13(Tamb)
  [Solar] -> Chart2/1(Solar)
  Chart2/1(FactorSolar) -> Switch19/3  "FactorSolar"
  Product/1 -> [sigSetTempZon1StC]
  [EXV2_Err] -> Logical Operator18/2
  [EXV1_Err] -> Logical Operator17/2
  Logical Operator16/1 -> Logical Operator18/1
  Logical Operator3/1 -> Logical Operator16/2
  Logical Operator12/1 -> Logical Operator8/11
  Logical Operator15/1 -> Logical Operator8/12
  [Tamb_Err] -> SensorErrorHandle12/2(SensorError)
  Tamb_Err/1 -> [Tamb_Err]
  Constant143/1 -> Thermal/163(KTHC_CompSpdmaxBC_rpm)
  [ErrCompForceOFF] -> Thermal/162(ErrCompForceOFF)
  [CompProEN] -> Logical Operator14/2
  [ErrCompForceOFF] -> Logical Operator14/1
  Logical Operator14/1 -> CompCtrl/11(CompProEN)
  Logical Operator13/1 -> [ErrAPTCForceOFF]
  [Blower_Err] -> Logical Operator13/1
  [AC] -> Thermal/22(AC)
  AC/1 -> [AC]
  [ErrEXV1FroceOFF] -> EXV1Ctrl/6(ErrEXV1FroceOFF)
  [ErrEXV2FroceOFF] -> EXV2Ctrl/6(ErrEXV2FroceOFF)
  SOTXV_Err/1 -> Logical Operator12/1
  Compare To Constant11/1 -> Logical Operator12/3
  Compare To Constant13/1 -> Logical Operator26/2
  Compare To Constant12/1 -> Logical Operator26/1
  Unit Delay8/1 -> Compare To Constant13/1, Compare To Constant12/1, Compare To Constant16/1
  [CabinMode] -> Unit Delay8/1
  [BatteryMode] -> Unit Delay7/1
  Unit Delay7/1 -> Compare To Constant11/1
  Logical Operator11/1 -> Logical Operator8/10
  Logical Operator10/1 -> Logical Operator11/1
  Logical Operator9/1 -> Logical Operator10/2
  Compare To Constant10/1 -> Logical Operator10/1
  Logical Operator5/1 -> Logical Operator6/2
  Logical Operator4/1 -> Logical Operator11/2, Logical Operator6/1
  NOT/1 -> Logical Operator9/1
  Unit Delay6/1 -> Compare To Constant9/1, Compare To Constant10/1
  Compare To Constant7/1 -> Logical Operator5/2
  Compare To Constant6/1 -> Logical Operator9/2, Logical Operator5/1
  Logical Operator7/1 -> NOT/1
  Logical Operator/1 -> Logical Operator8/9
  Comp_Err/1 -> Logical Operator8/8
  EXV2_Err/1 -> Logical Operator8/7, [EXV2_Err]
  EXV1_Err/1 -> Logical Operator8/6, [EXV1_Err]
  SOV3_Err/1 -> Logical Operator8/5
  SOV2_Err/1 -> Logical Operator8/4
  SOV1_Err/1 -> Logical Operator8/3
  PT_High_Tact_Err/1 -> Logical Operator8/2
  PT_High_P_Err/1 -> Logical Operator8/1
  Compare To Constant8/1 -> Logical Operator7/2
  Compare To Constant9/1 -> Logical Operator7/1
  Logical Operator6/1 -> Logical Operator17/1
  [ACSubMode] -> Unit Delay6/1
  [CabinMode] -> Unit Delay5/1
  Unit Delay5/1 -> Compare To Constant7/1, Compare To Constant8/1
  Unit Delay4/1 -> Compare To Constant6/1
  [BatteryMode] -> Unit Delay4/1
  PT_Low_T1_Err/1 -> Logical Operator4/2
  PT_Low_P1_Err/1 -> Logical Operator4/1
  PT_Low_T2_Err/1 -> Logical Operator1/2
  PT_Low_P2_Err/1 -> Logical Operator1/1
  Compare To Constant5/1 -> Logical Operator3/2
  Logical Operator2/1 -> Logical Operator3/1, Logical Operator15/1
  Compare To Constant4/1 -> Logical Operator2/2
  Compare To Constant3/1 -> Logical Operator2/1
  Logical Operator1/1 -> Logical Operator16/1, Logical Operator15/2
  Unit Delay3/1 -> Compare To Constant3/1, Compare To Constant4/1, Compare To Constant5/1
  [CabinMode] -> Unit Delay3/1
  [Blower_Err] -> Logical Operator/1
  Compare To Constant/1 -> Logical Operator/3
  Compare To Constant2/1 -> Logical Operator24/2
  Compare To Constant1/1 -> Logical Operator24/1
  Unit Delay/1 -> Compare To Constant1/1, Compare To Constant2/1, Compare To Constant15/1
  Unit Delay2/1 -> Compare To Constant/1
  [BatteryMode] -> Unit Delay2/1
  [CabinMode] -> Unit Delay/1
  Blower_Err/1 -> [Blower_Err]
  Constant142/1 -> WPTC/3(PresetValue)
  EWP3_Err/1 -> WPTC/2(EWP3_Err)
  [WPTC] -> WPTC/1(WPTC)
  Thermal/3(FrWPTCHeatPwr) -> [WPTC]  "FD_FrWPTCHeatPwr_Cmd"
  [AGS] -> RadiatorFan/3(AGS)
  AGS_Err/1 -> RadiatorFan/2(AGS_Err)
  [FAN] -> AGSandFan/3(FAN)
  Fan_Err/1 -> AGSandFan/2(Fan_Err)
  [FAN] -> RadiatorFan/1(FAN)
  [AGS] -> AGSandFan/1(AGSLV)
  Thermal/2(FAN) -> [FAN]
  Constant141/1 -> SensorErrorHandle11/3(PresetValue)
  Motor_Out_Temp_Err/1 -> SensorErrorHandle11/2(SensorError)
  Motor_Out_Temp/1 -> SensorErrorHandle11/1(DataIn)
  SensorErrorHandle11/1(DataOut) -> [Motor_Out_Temp]
  [TBMax] -> Subsystem2/3(TBMax)
  Motor_In_Temp_Err/1 -> Subsystem2/2(Motor_In_Temp_Err)
  Motor_In_Temp/1 -> Subsystem2/1(Motor_In_Temp)
  Subsystem2/1(Motor_In_TempFix) -> [Motor_In_Temp]
  [Motor_Out_Temp] -> Thermal/5(Motor_Out_Temp)
  [Motor_In_Temp] -> Thermal/4(Motor_In_Temp)
  Constant140/1 -> SensorErrorHandle10/3(PresetValue)
  SensorErrorHandle10/1(DataOut) -> [Bat_In_Temp]
  Bat_In_Temp_Err/1 -> SensorErrorHandle10/2(SensorError)
  Bat_In_Temp/1 -> SensorErrorHandle10/1(DataIn)
  Tincar_Err/1 -> Subsystem1/15(Tincar_Err)
  Tincar/1 -> Subsystem1/14(Tincar)
  [CabinMode] -> Subsystem1/13(CabinMode)
  Subsystem1/1(TincarFix) -> [Tincar]
  [T_Foot_Rr_Err] -> Subsystem1/12(T_Foot_Rr_Err)
  [T_Foot_Rr] -> Subsystem1/6(T_Foot_Rr)
  [T_Face_Rr] -> Subsystem1/5(T_Face_Rr)
  [T_Foot_R] -> Subsystem1/4(T_Foot_R)
  [T_Face_Rr_Err] -> Subsystem1/11(T_Face_Rr_Err)
  [T_Face_L] -> Subsystem1/1(T_Face_L)
  [T_Foot_R_Err] -> Subsystem1/10(T_Foot_R_Err)
  [T_Face_L_Err] -> Subsystem1/7(T_Face_L_Err)
  [T_Face_R] -> Subsystem1/2(T_Face_R)
  [T_Foot_L] -> Subsystem1/3(T_Foot_L)
  [T_Foot_L_Err] -> Subsystem1/9(T_Foot_L_Err)
  [T_Face_R_Err] -> Subsystem1/8(T_Face_R_Err)
  [T_Foot_Rr_Err] -> SensorErrorHandle9/2(SensorError)
  [T_Face_Rr_Err] -> SensorErrorHandle8/2(SensorError)
  [T_Foot_R_Err] -> SensorErrorHandle7/2(SensorError)
  [T_Foot_L_Err] -> SensorErrorHandle6/2(SensorError)
  [T_Face_R_Err] -> SensorErrorHandle5/2(SensorError)
  [T_Face_L_Err] -> SensorErrorHandle4/2(SensorError)
  SensorErrorHandle9/1(DataOut) -> [T_Foot_Rr]
  SensorErrorHandle8/1(DataOut) -> [T_Face_Rr]
  SensorErrorHandle7/1(DataOut) -> [T_Foot_R]
  SensorErrorHandle6/1(DataOut) -> [T_Foot_L]
  SensorErrorHandle5/1(DataOut) -> [T_Face_R]
  SensorErrorHandle4/1(DataOut) -> [T_Face_L]
  T_Foot_Rr/1 -> SensorErrorHandle9/1(DataIn)
  T_Face_Rr/1 -> SensorErrorHandle8/1(DataIn)
  T_Foot_R/1 -> SensorErrorHandle7/1(DataIn)
  T_Foot_L/1 -> SensorErrorHandle6/1(DataIn)
  T_Face_R/1 -> SensorErrorHandle5/1(DataIn)
  T_Face_L/1 -> SensorErrorHandle4/1(DataIn)
  Constant139/1 -> SensorErrorHandle9/3(PresetValue)
  Constant138/1 -> SensorErrorHandle8/3(PresetValue)
  Constant137/1 -> SensorErrorHandle7/3(PresetValue)
  Constant136/1 -> SensorErrorHandle6/3(PresetValue)
  Constant135/1 -> SensorErrorHandle5/3(PresetValue)
  Constant134/1 -> SensorErrorHandle4/3(PresetValue)
  T_Foot_Rr_Err/1 -> [T_Foot_Rr_Err]
  T_Face_Rr_Err/1 -> [T_Face_Rr_Err]
  T_Foot_R_Err/1 -> [T_Foot_R_Err]
  T_Foot_L_Err/1 -> [T_Foot_L_Err]
  T_Face_R_Err/1 -> [T_Face_R_Err]
  T_Face_L_Err/1 -> [T_Face_L_Err]
  [T_Foot_Rr] -> APTC/11(T_Foot_Rr)
  [T_Face_Rr] -> APTC/10(T_Face_Rr)
  [T_Foot_R] -> APTC/9(T_Foot_R)
  [T_Foot_L] -> APTC/8(T_Foot_L)
  [T_Face_R] -> APTC/7(T_Face_R)
  [T_Face_L] -> APTC/6(T_Face_L)
  [Tevap] -> Thermal/16(Tevap)
  SensorErrorHandle3/1(DataOut) -> [Tevap]
  Constant133/1 -> SensorErrorHandle3/3(PresetValue)
  Tevap_Err/1 -> SensorErrorHandle3/2(SensorError)
  Tevap/1 -> SensorErrorHandle3/1(DataIn)
  SensorErrorHandle2/1(DataOut) -> Add1/2
  SensorErrorHandle1/1(DataOut) -> Add1/1
  Constant132/1 -> SensorErrorHandle2/3(PresetValue)
  SolarR/1 -> SensorErrorHandle2/1(DataIn)
  SolarR_Err/1 -> SensorErrorHandle2/2(SensorError)
  Constant131/1 -> SensorErrorHandle1/3(PresetValue)
  SolarL_Err/1 -> SensorErrorHandle1/2(SensorError)
  SolarL/1 -> SensorErrorHandle1/1(DataIn)
  Constant130/1 -> SensorErrorHandle12/3(PresetValue)
  Tamb/1 -> SensorErrorHandle12/1(DataIn)
  SensorErrorHandle12/1(DataOut) -> [Tamb]
  Constant129/1 -> Thermal/161(KTHC_TDcChgBC_C)
  [EXVOpen] -> EXV2Ctrl/5(EXVOpen)
  [EXVOpen] -> EXV1Ctrl/5(EXVOpen)
  Subsystem/5(EXVOpen) -> [EXVOpen]
  EACProtectEnable/1 -> Thermal/160(EACProtectEnable)
  PET/1 -> Thermal/159(PET)
  Thermal/19(dy) -> Scope/1
  Rr_LLCTemp/1 -> Thermal/158(Rr_LLCTemp)
  Fr_LLCTemp/1 -> Thermal/157(Fr_LLCTemp)
  Constant128/1 -> Thermal/156(KTHC_T5MinLLC_C)
  Constant127/1 -> Thermal/155(KTHC_T4MaxLLC_C)
  Constant126/1 -> Thermal/154(KTHC_T4MinLLC_C)
  Constant125/1 -> Thermal/153(KTHC_T3MaxLLC_C)
  Constant124/1 -> Thermal/152(KTHC_T3MinLLC_C)
  Constant123/1 -> Thermal/151(KTHC_T2MaxLLC_C)
  Constant122/1 -> Thermal/150(KTHC_T2MinLLC_C)
  Constant121/1 -> Thermal/149(KTHC_T1MaxLLC_C)
  Thermal/12(SOTXV) -> [SOTXV]
  Constant118/1 -> Chart/4(KTHC_CompSotxvOp_K)
  Constant120/1 -> Chart/6(KTHC_SotxvProLo_kPa)
  Constant117/1 -> Chart/3(KTHC_CompSotxvOpLow_rpm)
  Constant119/1 -> Chart/5(KTHC_SotxvProHi_kPa)
  Subsystem/1(FD_Comp_Cmd) -> Chart/2(CompIn)
  [CabinMode] -> Chart/1(CabinMode)
  Chart/2(SOTXVout) -> FD_SOTXV_Cmd/1
  [PT_High_P] -> Chart/7(PT_High_P)
  [SOTXV] -> Chart/8(SOTXV)
  Constant116/1 -> Thermal/148(KTHC_tb_K)
  Constant115/1 -> Thermal/147(KTHC_ta_K)
  Constant114/1 -> Thermal/146(KTHC_bDeice_K)
  Constant113/1 -> Thermal/145(KTHC_aDeice_K)
  Constant112/1 -> Thermal/144(KTHC_TwOhtOn_C)
  Constant111/1 -> Thermal/143(KTHC_TwOhtOff_C)
  Constant110/1 -> Thermal/142(KTHC_TimeDeiceMax_K)
  Constant109/1 -> Thermal/141(KTHC_Time0_K)
  Constant108/1 -> Thermal/140(KTHC_TambHPmin_C)
  Constant107/1 -> Thermal/139(KTHC_TDeice2_C)
  Constant106/1 -> Thermal/138(KTHC_TDeice1_C)
  Constant105/1 -> Thermal/136(KTHC_PDeiceMax_kPa)
  Constant104/1 -> Thermal/135(KTHC_DeiceCycTime_K)
  Constant103/1 -> Thermal/134(KTHC_CompMinDeice_rpm)
  Constant102/1 -> Thermal/133(KTHC_CompMaxDeice_rpm)
  Bat_Out_Temp/1 -> Thermal/132(Bat_Out_Temp)
  [PwrSta] -> Thermal/7(PwrSta)
  [dAy] -> Thermal/131(dAy)
  1-D Lookup Table/1 -> [dAy]
  [Tamb] -> 1-D Lookup Table/1
  APTC/3(FD_FrRiAPTCHeatPwr_Cmd) -> FD_FrRiAPTCHeatPwr_Cmd/1  "FD_FrRiAPTCHeatPwr_Cmd"
  Switch11/1 -> FD_RrAPTCHeatPwr_Cmd/1  "FD_RrAPTCHeatPwr_Cmd"
  APTC/2(FD_FrLeAPTCHeatPwr_Cmd) -> FD_FrLeAPTCHeatPwr_Cmd/1  "FD_FrLeAPTCHeatPwr_Cmd"
  [VehSpeed] -> APTC/4(VehSpeed)
  [VehSpeed] -> Thermal/20(VehSpeed)
  Constant96/1 -> Thermal/130(KTHC_DehumidityEN_flg)
  Constant100/1 -> Thermal/129(KTHC_Tdeheat2_C)
  Constant99/1 -> Thermal/128(KTHC_Tdeheat1_C)
  Constant98/1 -> Thermal/127(KTHC_Tdefog_C)
  Constant97/1 -> Thermal/126(KTHC_TimeD_K)
  Constant95/1 -> Thermal/125(KTHC_ThiDehum_C)
  Constant94/1 -> Thermal/124(KTHC_PhiDehum_kPa)
  Constant93/1 -> Thermal/123(KTHC_CompSpdmid_rpm)
  Constant92/1 -> Thermal/122(KTHC_APTCQminRe_W)
  Constant91/1 -> Thermal/121(KTHC_Twmset_C)
  Constant90/1 -> Thermal/120(KTHC_Tambset_C)
  Constant89/1 -> Thermal/119(KTHC_DTh1_C)
  Constant88/1 -> Thermal/118(KTHC_Plow2Setpoint_kPa)
  Constant87/1 -> Thermal/117(KTHC_CompSpdmin_rpm)
  Constant86/1 -> Thermal/116(KTHC_Timewcd_K)
  Constant85/1 -> Thermal/115(KTHC_T3winSetpointBC_C)
  Constant84/1 -> Thermal/114(KTHC_TBPmin_C)
  Constant83/1 -> Thermal/113(KTHC_TBPmax_C)
  Constant82/1 -> Thermal/112(KTHC_CompSpdmax_rpm)
  Constant81/1 -> Thermal/111(KTHC_DTwBBin_C)
  Constant80/1 -> Thermal/110(KTHC_DTwBMoin2_C)
  Constant79/1 -> Thermal/109(KTHC_DTwBMoin1_C)
  Constant78/1 -> Thermal/91(KTHC_T2MaxBH_C)
  Constant77/1 -> Thermal/90(KTHC_T1MinBH_C)
  Constant75/1 -> Thermal/108(KTHC_TWinmin_C)
  Constant74/1 -> Thermal/107(KTHC_TWinmax_C)
  Constant65/1 -> Thermal/97(KTHC_T5MaxBH_C)
  Constant64/1 -> Thermal/96(KTHC_T4MinBH_C)
  Constant63/1 -> Thermal/95(KTHC_T4MaxBH_C)
  Constant62/1 -> Thermal/94(KTHC_T3MinBH_C)
  Constant61/1 -> Thermal/93(KTHC_T3MaxBH_C)
  Constant60/1 -> Thermal/92(KTHC_T2MinBH_C)
  Constant59/1 -> Thermal/89(KTHC_VehSdAGSCtrl_kph)
  Constant58/1 -> Thermal/88(KTHC_VehSdAGS100_kph)
  Constant57/1 -> Thermal/87(KTHC_VehSdFanOff_kph)
  Constant56/1 -> Thermal/86(KTHC_VehSdFanOn_kph)
  Constant55/1 -> Thermal/85(KTHC_DTambSat_C)
  Constant54/1 -> Thermal/84(KTHC_TwRcolOff_C)
  Constant53/1 -> Thermal/83(KTHC_TwRcolOn_C)
  Constant52/1 -> Thermal/82(KTHC_TWVRcolPos_pct)
  Constant50/1 -> Thermal/81(KTHC_P5MaxLo_kPa)
  Constant49/1 -> Thermal/80(KTHC_P4MinLo_kPa)
  Constant48/1 -> Thermal/79(KTHC_P4MaxLo_kPa)
  Constant47/1 -> Thermal/78(KTHC_P3MinLo_kPa)
  Constant46/1 -> Thermal/77(KTHC_P3MaxLo_kPa)
  Constant51/1 -> Thermal/76(KTHC_P2MinLo_kPa)
  Constant44/1 -> Thermal/75(KTHC_P5MinHi_kPa)
  Constant43/1 -> Thermal/74(KTHC_P4MaxHi_kPa)
  Constant42/1 -> Thermal/73(KTHC_P4MinHi_kPa)
  Constant41/1 -> Thermal/72(KTHC_P3MaxHi_kPa)
  Constant40/1 -> Thermal/71(KTHC_P3MinHi_kPa)
  Constant45/1 -> Thermal/70(KTHC_P2MaxHi_kPa)
  Constant37/1 -> Thermal/69(KTHC_T5MinMT_C)
  Constant36/1 -> Thermal/68(KTHC_T4MaxMT_C)
  Constant35/1 -> Thermal/67(KTHC_T4MinMT_C)
  Constant34/1 -> Thermal/66(KTHC_T3MaxMT_C)
  Constant33/1 -> Thermal/65(KTHC_T3MinMT_C)
  Constant39/1 -> Thermal/64(KTHC_T2MaxMT_C)
  Constant38/1 -> Thermal/63(KTHC_T2MinMT_C)
  Constant32/1 -> Thermal/62(KTHC_T1MaxMT_C)
  Constant29/1 -> Thermal/61(KTHC_T5MinMCU_C)
  Constant28/1 -> Thermal/60(KTHC_T4MaxMCU_C)
  Constant27/1 -> Thermal/59(KTHC_T4MinMCU_C)
  Constant26/1 -> Thermal/58(KTHC_T3MaxMCU_C)
  Constant25/1 -> Thermal/57(KTHC_T3MinMCU_C)
  Constant31/1 -> Thermal/56(KTHC_T2MaxMCU_C)
  Constant30/1 -> Thermal/55(KTHC_T2MinMCU_C)
  Constant24/1 -> Thermal/54(KTHC_T1MaxMCU_C)
  Constant21/1 -> Thermal/53(KTHC_T5MinCCU_C)
  Constant20/1 -> Thermal/52(KTHC_T4MaxCCU_C)
  Constant19/1 -> Thermal/51(KTHC_T4MinCCU_C)
  Constant18/1 -> Thermal/50(KTHC_T3MaxCCU_C)
  Constant17/1 -> Thermal/49(KTHC_T3MinCCU_C)
  Constant23/1 -> Thermal/48(KTHC_T2MaxCCU_C)
  Constant22/1 -> Thermal/47(KTHC_T2MinCCU_C)
  Constant16/1 -> Thermal/46(KTHC_T1MaxCCU_C)
  Constant15/1 -> Thermal/45(KTHC_T5MinBC_C)
  Constant14/1 -> Thermal/44(KTHC_T4MaxBC_C)
  Constant12/1 -> Thermal/43(KTHC_T4MinBC_C)
  Constant11/1 -> Thermal/42(KTHC_T3MaxBC_C)
  Constant10/1 -> Thermal/41(KTHC_T3MinBC_C)
  Constant9/1 -> Thermal/40(KTHC_T2MaxBC_C)
  Constant8/1 -> Thermal/39(KTHC_T2MinBC_C)
  Constant/1 -> Thermal/38(KTHC_T1MaxBC_C)
  [PwrSta] -> BlowerCtrl/12(PwrSta)
  [PT_High_P] -> CompCtrl/12(PT_High_P)
  Constant7/1 -> Thermal/37(APTCQminD)
  [ACSubMode] -> BlowerCtrl/11(ACSubMode)
  WaterFillReq/1 -> Thermal/36(WaterFillReq)
  PT_High_Tact/1 -> Thermal/26(PT_High_T)
  [DfrstReq] -> Thermal/35(DfrstReq)
  [DfrstReq] -> BlowerCtrl/10(DfrstReq)
  DfrstReq/1 -> [DfrstReq]
  [sigSetTempZon1StC] -> Thermal/23(sigSetTempZon1StC)
  AGSandFan/1(AGSOut) -> FD_AGS_Cmd/1  "FD_AGS_Cmd"
  RadiatorFan/1(CoolgFanActDuty) -> CoolgFanActDuty/1  "CoolgFanActDuty"
  Subsystem3/5(EWP3) -> FD_EWP3_Cmd/1  "FD_EWP3_Cmd"
  Thermal/9(EWP2) -> EWP3/1(EWPLV)
  Thermal/8(EWP1) -> EWP1/1(EWPLV)
  Constant6/1 -> Thermal/34(Tdeice)
  Constant5/1 -> Thermal/33(Tice)
  Constant3/1 -> Thermal/32(Timehu2)
  Constant2/1 -> Thermal/31(Timehu1)
  Constant4/1 -> EXV2Ctrl/1(EXV2SHSetpoint)
  Thermal/16(BatteryMode) -> BatteryMode/1, [BatteryMode]
  Thermal/17(CabinMode) -> [CabinMode], CabinMode/1
  VSCP_AGSCloseSta_flg/1 -> Thermal/28(VSCP_AGSCloseSta_flg)
  [CompFB] -> Subsystem/3(CompFB)
  EXV1Ctrl/1(EXV1) -> FD_EXV1_Cmd/1  "FD_EXV1_Cmd"
  Constant13/1 -> EXV1Ctrl/1(EXV1SHSetpoint)
  HVBMTempMax/1 -> [TBMax]
  PT_Low_P2/1 -> [PT_Low_P2]
  Subsystem/2(FD_SOV1_Cmd) -> FD_SOV1_Cmd/1
  PT_ Low_T1/1 -> EXV1Ctrl/3(PT_ Low_T1)
  [TBMax] -> CompCtrl/5(TBMax)
  PT_High_P/1 -> [PT_High_P]
  Subsystem/4(FD_SOV3_Cmd) -> FD_SOV3_Cmd/1
  Add1/1 -> Gain2/1
  Subsystem/3(FD_SOV2_Cmd) -> FD_SOV2_Cmd/1
  PT_ Low_P1/1 -> [PT_Low_P1]
  HVBMTempMin/1 -> Thermal/9(TBMin)
  Thermal/4(BattPump3) -> EWP2/1(EWPLV)
  PwrSta/1 -> [PwrSta]
  [sigSetTempZon1St] -> BlowerCtrl/2(sigSetTempZon1St)
  [sigSetTempZon1St] -> CompCtrl/2(sigSetTempZon1St)
  PT_ Low_T2/1 -> EXV2Ctrl/2(PT_ Low_T2)
  [CompPID] -> CompCtrl/1(CompPIDin)
  Thermal/13(TWV) -> [TWV1in]
  sigAirIntenZon1St/1 -> [sigAirIntenZon1St]
  EXV2Ctrl/2(Tsat_low2) -> [Tsat_low2]  "Tsat_low2"
  [Tincar] -> BlowerCtrl/4(Tincar)
  [PT_Low_P2] -> Thermal/6(PT_Low_P2)
  [sigSetTempZon1StC] -> CompCtrl/3(sigSetTempZon1StC)
  EXV2Ctrl/1(EXV2) -> FD_EXV2_Cmd/1  "FD_EXV2_Cmd"
  [PT_Low_P1] -> EXV1Ctrl/2(PT_ Low_P1)
  Chart/1(CompOut) -> FD_Comp_Cmd/1
  [CompFB] -> CompCtrl/9(CompFB)
  [CompSpd] -> Subsystem/1(CompSpd)
  ACAuto/1 -> [ACAuto]
  CompFB/1 -> [CompFB]
  [CabinMode] -> Subsystem/2(CabinMode)
  CompProEN/1 -> [CompProEN]
  CompCtrl/1(CompSpd) -> [CompSpd]
  [sigAirIntenZon1St] -> BlowerCtrl/6(sigAirIntenZon1St)
  BlowerCtrl/1(VTHC_FDBlowerCmd_pct) -> FD_Blower_Cmd/1  "FD_Blower_Cmd"
  [ACAuto] -> BlowerCtrl/5(ACAuto)
  [Tamb] -> BlowerCtrl/7(Tamb)
  [sigSetTempZon1StC] -> BlowerCtrl/3(sigSetTempZon1StC)
  [Tincar] -> CompCtrl/4(Tincar)
  [BlowerPID] -> BlowerCtrl/1(BlowerPID)
  [Bat_In_Temp] -> CompCtrl/6(Bat_In_Temp)
  [PT_Low_P2] -> CompCtrl/7(PT_Low_P2)
  Constant1/1 -> CompCtrl/8(PT_ Low_P2Setpoint)
  [CompSet] -> CompCtrl/10(CompSet)
  Gain2/1 -> [Solar]
  [Blowersolar] -> BlowerCtrl/8(Blowersolar)
  [CabinMode] -> BlowerCtrl/9(CabinMode)
  [EXV2PIDMode] -> EXV2Ctrl/4(EXV2PIDMode)  "EXV2PIDMode"
  [PT_Low_P2] -> EXV2Ctrl/3(PT_ Low_P2)
  APTC/1(APTCQ) -> Unit Delay1/1
  Unit Delay1/1 -> [APTCQ]
  [APTCPID] -> APTC/3(APTCPID)
  [Tincar] -> APTC/2(Tincar)
  [sigSetTempZon1St] -> APTC/1(sigSetTempZon1St)
  [BatteryMode] -> EXV1Ctrl/4(BatteryMode)
  [Bat_In_Temp] -> Thermal/2(Bat_In_Temp)
  Rr_MCUTemp/1 -> Thermal/12(TRrMCU)
  [CompFB] -> Thermal/3(CompSpd)
  [Tsat_low2] -> Thermal/19(Tsat_low2)
  VehSpeed/1 -> [VehSpeed]
  CompCtrl/6(VTHC_Compe_K) -> VTHC_Compe_K/1  "VTHC_Compe_K"
  [sigSetTempZon1St] -> Thermal/21(sigSetTempZon1St)
  [TBMax] -> Thermal/8(TBMax)
  Thermal/14(APTCPID) -> [APTCPID]
  BlowerCtrl/2(VTHC_Blowere_K) -> VTHC_Blowere_K/1  "VTHC_Blowere_K"
  Thermal/6(CompPID) -> [CompPID]
  EXV2Ctrl/5(VTHC_EXV2U_K) -> VTHC_EXV2U_K/1  "VTHC_EXV2U_K"
  Rr_TMTemp/1 -> Thermal/13(TRrTM)
  Thermal/18(EDriveMode) -> EDriveMode/1
  APTC/8(VTHC_APTCe_K) -> VTHC_APTCe_K/1  "VTHC_APTCe_K"
  Thermal/5(BlowerPID) -> [BlowerPID]
  [PT_High_P] -> Thermal/24(ACHP)
  [PT_Low_P2] -> Thermal/25(ACLP)
  Fr_MCUTemp/1 -> Thermal/10(TFrMCU)
  WPTC/1(DataOut) -> FD_FrWPTCHeatPwr_Cmd/1  "FD_FrWPTCHeatPwr_Cmd"
  BlowerCtrl/3(VTHC_BlowerP_K) -> VTHC_BlowerP_K/1  "VTHC_BlowerP_K"
  CompCtrl/5(VTHC_CompDeltaU_K) -> VTHC_CompDeltaU_K/1  "VTHC_CompDeltaU_K"
  Fr_TMTemp/1 -> Thermal/11(TFrTM)
  EXV1Ctrl/4(VTHC_EXV1U_K) -> VTHC_EXV1U_K/1  "VTHC_EXV1U_K"
  DCDCTemp/1 -> Thermal/15(Tdcdc)
  CompCtrl/4(VTHC_CompU_K) -> VTHC_CompU_K/1  "VTHC_CompU_K"
  BlowerCtrl/6(VTHC_Vbase_pct) -> VTHC_Vbase_pct/1  "VTHC_Vbase_pct"
  EXV2Ctrl/3(VTHC_EXV2P_K) -> VTHC_EXV2P_K/1  "VTHC_EXV2P_K"
  OBCTemp/1 -> Thermal/18(Tobc)
  [Tamb] -> Thermal/14(Tamb)
  Thermal/11(FWV) -> [FWV1in]
  EXV1Ctrl/3(VTHC_EXV1I_K) -> VTHC_EXV1I_K/1  "VTHC_EXV1I_K"
  Thermal/7(CompSet) -> [CompSet]
  Subsystem3/3(EWP1) -> FD_EWP1_Cmd/1  "FD_EWP1_Cmd"
  EXV1Ctrl/2(VTHC_EXV1P_K) -> VTHC_EXV1P_K/1  "VTHC_EXV1P_K"
  CompCtrl/3(VTHC_CompI_K) -> VTHC_CompI_K/1  "VTHC_CompI_K"
  EXV2Ctrl/6(VTHC_EXV2e_K) -> VTHC_EXV2e_K/1  "VTHC_EXV2e_K"
  EXV1Ctrl/5(VTHC_EXV1e_K) -> VTHC_EXV1e_K/1  "VTHC_EXV1e_K"
  EXV2Ctrl/4(VTHC_EXV2I_K) -> VTHC_EXV2I_K/1  "VTHC_EXV2I_K"
  BlowerCtrl/5(VTHC_BlowerU_K) -> VTHC_BlowerU_K/1  "VTHC_BlowerU_K"
  [APTCQ] -> Thermal/27(APTCQ)
  [Tincar] -> Thermal/17(Tincar)
  CompCtrl/2(VTHC_CompP_K) -> VTHC_CompP_K/1  "VTHC_CompP_K"
  BlowerCtrl/4(VTHC_BlowerI_K) -> VTHC_BlowerI_K/1  "VTHC_BlowerI_K"
  APTC/6(VTHC_APTCI_K) -> VTHC_APTCI_K/1  "VTHC_APTCI_K"
  Thermal/10(EXV2PIDMode) -> [EXV2PIDMode]
  APTC/7(VTHC_APTCU_K) -> VTHC_APTCU_K/1  "VTHC_APTCU_K"
  Thermal/15(ACSubMode) -> [ACSubMode], ACSubMode/1
  APTC/5(VTHC_APTCP_K) -> VTHC_APTCP_K/1  "VTHC_APTCP_K"
  ShiftGearPosn/1 -> Thermal/29(ShiftGearPosn)
  Switch7/1 -> Add2/2
  Constant235/1 -> Switch7/1
  Constant236/1 -> Switch7/3
  Add2/1 -> Switch8/1
  [PwrSta] -> Relational Operator7/1
  Constant237/1 -> Switch8/3
  Logical Operator31/1 -> Switch7/2, Logical Operator35/2
  Logical Operator35/1 -> Switch8/2
  Relational Operator7/1 -> Logical Operator35/1
  Constant238/1 -> Relational Operator7/2
  Compare To Constant19/1 -> [APTCForceOFF], VTHC_FDCTHCMAPTCForceOFFSta_flg/1
  Unit Delay11/1 -> Add2/1
  Constant239/1 -> Switch9/1
  Switch9/1 -> Unit Delay11/1, Compare To Constant19/1
  APTCFailDTC/1 -> Switch9/2
  Switch8/1 -> Saturation1/1
  Saturation1/1 -> Switch9/3
  APTC/4(FD_RrAPTCHeatPwr_Cmd) -> Switch11/1  "FD_RrAPTCHeatPwr_Cmd"
  Constant244/1 -> Switch11/3
  ChrgPlugSta/1 -> [ChrgPlugSta]
  [ChrgPlugSta] -> Thermal/30(ChrgPlugSta)
  [ChrgPlugSta] -> Compare To Constant18/1
  Compare To Constant18/1 -> Logical Operator31/3
  VINP_HVBattSOC_pct/1 -> Thermal/210(VINP_HVBattSOC_pct)
  VINP_IVIWPTCSWSta_flg/1 -> Thermal/211(VINP_IVIWPTCSWSta_flg)
  Thermal/20(VTHC_FDCTHCMPreWPTCHeatSta_enum) -> Unit Delay10/1, VTHC_FDCTHCMPreWPTCHeatSta_enum/1
  RrAPTCEN/1 -> [RrAPTCEN]
  [RrAPTCEN] -> Switch11/2
  sigWindDirZon1St/1 -> BlowerCtrl/13(sigWindDirZon1St)
  [RrAPTCEN] -> BlowerCtrl/14(RrAPTCEN)
  Constant101/1 -> Switch5/1
  Constant229/1 -> Switch5/3
  Switch5/1 -> [T1MinBAH]
  [ChargeReq] -> Switch5/2
  [T1MinBAH] -> Thermal/137(T1MinBAH)
  [ChargeReq] -> Switch6/2
  Switch6/1 -> [T2MinBAH]
  Constant231/1 -> Switch6/3
  Constant230/1 -> Switch6/1
  [T2MinBAH] -> Thermal/99(T2MinBAH)
  Constant70/1 -> Switch10/1
  Constant240/1 -> Switch10/3
  Switch10/1 -> [T2MaxBAH]
  [ChargeReq] -> Switch10/2
  [T2MaxBAH] -> Thermal/98(T2MaxBAH)
  Constant67/1 -> Switch12/1
  Constant232/1 -> Switch12/3
  Switch12/1 -> [T3MaxBAH]
  [ChargeReq] -> Switch12/2
  [T3MaxBAH] -> Thermal/100(T3MaxBAH)
  [ChargeReq] -> Switch13/2
  Switch13/1 -> [T3MinBAH]
  Constant66/1 -> Switch13/3
  Constant68/1 -> Switch13/1
  [T3MinBAH] -> Thermal/101(T3MinBAH)
  Constant69/1 -> Switch14/1
  Constant241/1 -> Switch14/3
  Switch14/1 -> [T4MaxBAH]
  [ChargeReq] -> Switch14/2
  [T4MaxBAH] -> Thermal/102(T4MaxBAH)
  [ChargeReq] -> Switch15/2
  Switch15/1 -> [WPTCBAH1]
  Constant243/1 -> Switch15/3
  Constant71/1 -> Switch15/1
  Constant73/1 -> Switch16/1
  Constant72/1 -> Switch16/3
  Switch16/1 -> [WPTCBAH2]
  [ChargeReq] -> Switch16/2
  [ChargeReq] -> Switch17/2
  Switch17/1 -> [WPTCBAH3]
  Constant76/1 -> Switch17/3
  Constant242/1 -> Switch17/1
  Constant245/1 -> Switch18/1
  Constant246/1 -> Switch18/3
  Switch18/1 -> [WPTCBAH4]
  [ChargeReq] -> Switch18/2
  [WPTCBAH4] -> Thermal/106(LevelWPTCBAH4)
  [WPTCBAH3] -> Thermal/105(LevelWPTCBAH3)
  [WPTCBAH2] -> Thermal/104(LevelWPTCBAH2)
  [WPTCBAH1] -> Thermal/103(LevelWPTCBAH1)
  Unit Delay10/1 -> [FDCTHCMPreWPTCHeatSta]
  [ChrgPlugSta] -> Compare To Constant20/1
  [FDCTHCMPreWPTCHeatSta] -> Compare To Constant21/1
  Compare To Constant20/1 -> Logical Operator32/1
  Compare To Constant21/1 -> Logical Operator32/2
  Logical Operator32/1 -> [ChargeReq]
  EWP2/1(EWPOut) -> [EWP3in]
  [EWP3in] -> Subsystem3/5(EWP3in)
  EWP1/1(EWPOut) -> [EWP1in]
  [EWP1in] -> Subsystem3/3(EWP1in)
  Subsystem3/4(EWP2) -> FD_EWP2_Cmd/1  "FD_EWP2_Cmd"
  EWP3/1(EWPOut) -> [EWP2in]  "FD_EWP2_Cmd"
  [EWP2in] -> Subsystem3/4(EWP2in)
  Subsystem3/1(FWV) -> FD_FWV_Cmd/1  "FD_FWV_Cmd"
  [FWV1in] -> Subsystem3/1(FWVin)
  Subsystem3/2(TWV) -> FD_TWV_Cmd/1  "FD_TWV_Cmd"
  [TWV1in] -> Subsystem3/2(TWVin)
  Constant247/1 -> Subsystem3/6(BalanceSW)
  Constant248/1 -> Thermal/212(KTHC_DTwBMoin3_C)
  Switch19/1 -> Product/2
  Subsystem4/1(HeatReq) -> Switch19/2
  Constant249/1 -> Switch19/1
  [Tamb] -> Subsystem4/2(Tamb)
  Constant250/1 -> Thermal/213(KTHC_ForceLeaveCool_C)
  Constant251/1 -> Thermal/214(KTHC_ForceLeaveHeat_C)
